simulink model "r_LIC"  (R2018a)
settings: Solver=VariableStepAuto  StartTime=0.0  StopTime=10.0  RelTol=1e-3
undefined symbols (not defined in the file): Q_i_A, Q_i_G
settings Model: Creator=cgonterman  LastModifiedBy=cgonterman

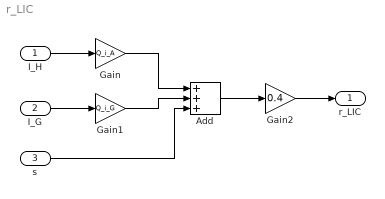
== system r_LIC ==
  "I_H " : Inport
  I_G : Inport  Port=2
  s : Inport  Port=3
  Add : Sum  Inputs=+++
  Gain : Gain  Gain=Q_i_A
  Gain1 : Gain  Gain=Q_i_G
  Gain2 : Gain  Gain=0.4
  "r_LIC " : Outport
  wires:
  "I_H "/1 -> Gain/1
  I_G/1 -> Gain1/1
  Gain/1 -> Add/1
  Gain1/1 -> Add/2
  s/1 -> Add/3
  Add/1 -> Gain2/1
  Gain2/1 -> "r_LIC "/1
